simulink model "localizeUsingLidar"  (R2023b)
settings: Solver=VariableStepAuto  StartTime=0.0  StopTime=28.964  RelTol=1e-3
PreLoadFcn:
  | data = load('ReferencePathForward.mat');
  | 
  | refPosesX = data.ReferencePathForward.refPosesX;
  | refPosesY = data.ReferencePathForward.refPosesY;
  | refPosesT = data.ReferencePathForward.refPosesT;
  | 
  | load('parkingLotPCMapPoints.mat','ptCloudMapPoints');
model workspace (MAT data in the model file):
  ndtMap = pcmapndt
  ndtMap.any.SelectedSubmap = [-73.8227987289 40.1600699425 -29.3149013519 63.6737504005 0.110943684975 6.5344303928]
  ndtMap.any.XLimits = [-73.8227987289 40.1600699425]
  ndtMap.any.YLimits = [-29.3149013519 63.6737504005]
  ndtMap.any.ZLimits = [0.110943684975 6.5344303928]
  ndtMap.any.VoxelSize = 1
  ndtMap.any.VoxelMean = [-5.69730867658 -5.01883643014 -68.9383283343 -43.7471444266 11.2284455981 12.0427000258 13.2013916016 14.026733126 -69.7659169977 -45.9612937927 -43.6656163534 -18.7063802083 ... (31146 elements, 10382x3)]
  ndtMap.any.VoxelCovariance = [0.0677527841433 0.0204767959446 0.0010976444077 0.0204767959445 0.0285064886293 0.00050731343504 0.0010976444077 0.000507313435039 0.000784462408784 0.0377123915766 -0.00599493818508 0.000197123956374 ... (93438 elements, 3x3x10382)]
  ndtMap.any.VoxelInverseCovariance = [19.1019935486 -13.3999087348 -18.0623602948 -13.3999087348 44.8881032169 -10.2796550333 -18.0623602948 -10.2796550332 1306.67963741 55.6473126486 182.683156062 -17.3445014094 ... (93438 elements, 3x3x10382)]
  ndtMap.any.VoxelNumPoints = [7 7 7 7 7 9 20 14 11 10 6 12 ... (10382 elements, 10382x1)]
  ndtMap.any.Version = 1
undefined symbols (not defined in the file or in its folder): ptCloudMapPoints
libraries: sim3dautolib x36, sim3dphyssensorlib x1, sim3dlib x1
settings Model: Creator=The MathWorks, Inc.  LastModifiedBy=mahi1
settings SolverCC: AlgebraicLoopSolver=TrustRegion  MaxZcPerStep=1
settings DebuggingCC: UnconnectedInputMsg=warning  UnconnectedOutputMsg=warning  UnconnectedLineMsg=warning
settings ModelReferenceCC: EnableRefExpFcnMdlSchedulingChecks=on
settings RTWCC: DLArmComputeVersion=19.05

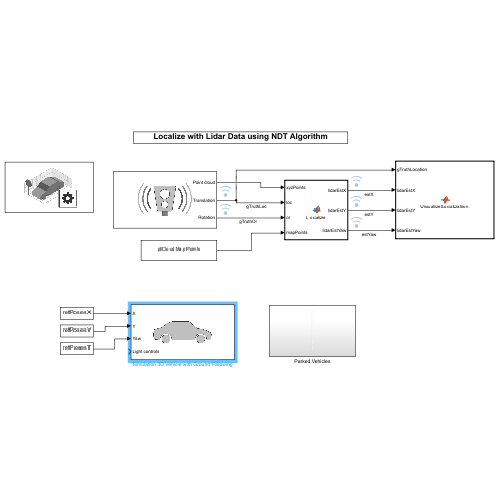
[thumbnail: Simulink's stored preview of the top-level diagram]
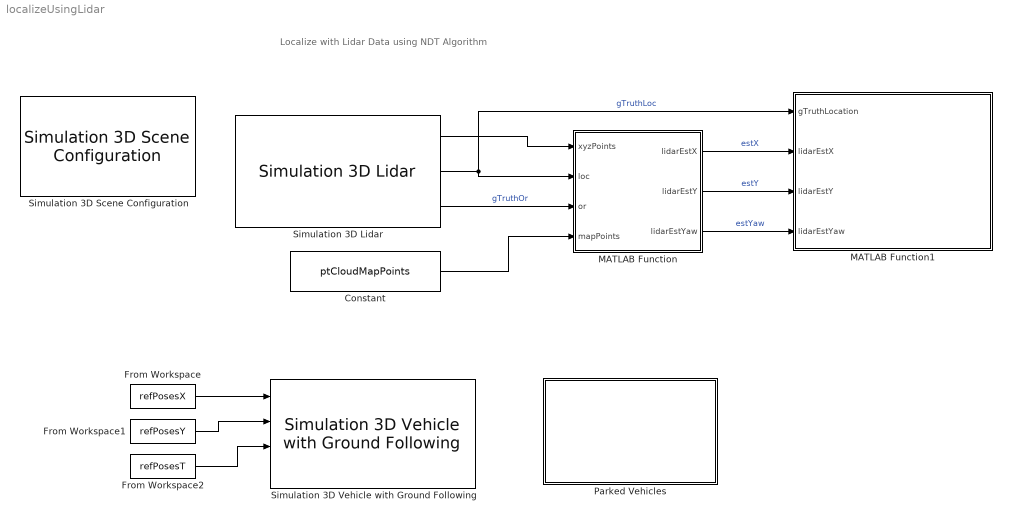
== system localizeUsingLidar ==
  note: Localize with Lidar Data using NDT Algorithm
  Constant : Constant  Value=ptCloudMapPoints
  From Workspace : FromWorkspace  VariableName=refPosesX  OutputAfterFinalValue=Holding final value
  From Workspace1 : FromWorkspace  VariableName=refPosesY  OutputAfterFinalValue=Holding final value
  From Workspace2 : FromWorkspace  VariableName=refPosesT  OutputAfterFinalValue=Holding final value
  MATLAB Function : MATLAB Function  TreatAsAtomicUnit=on
  MATLAB Function1 : MATLAB Function  StopFcn=|  TreatAsAtomicUnit=on
      | % Find figure by name
      | viewerFigure = findall(groot, 'type', 'figure', ...
      |     'name','Scene Map Display');
      | 
      | % Close figure
      | if ~isempty(viewerFigure)
      |     viewerFigure = viewerFigure(end);
      |     if isvalid(viewerFigure)
      |         close(viewerFigure);
      |     end
      | end
  Parked Vehicles : Subsystem
  Simulation 3D Lidar : sim3dphyssensorlib/Simulation 3D Lidar  Priority=1  sensorTag=Sim3dSensor1  sensorId=1  sensorName=Sim3dSensor1  vehTagList={'Scene Origin';'SimulinkVehicle1';'SimulinkVehicle10';'SimulinkVehicle11';'SimulinkVehicle12';'SimulinkVehicle13';'SimulinkVehicle14';'SimulinkVehicle15';'SimulinkVehicle16';'SimulinkVehicle17';'SimulinkVehicle18';'SimulinkVehicle19';'SimulinkVehicle2';'SimulinkVehicle20';'SimulinkVehicle21';'SimulinkVehicle22';'SimulinkVehicle23';'SimulinkVehicle24';'SimulinkVehicle25';'SimulinkVehicle26';'SimulinkVehicle27';'SimulinkVehicle28';'SimulinkVehicle29';'SimulinkVehicle3';'SimulinkVehicle30';'SimulinkVehicle31';'SimulinkVehicle32';'SimulinkVehicle33';'SimulinkVehicle34';'SimulinkVehicle35';'SimulinkVehicle36';'SimulinkVehicle4';'SimulinkVehicle5';'SimulinkVehicle6';'SimulinkVehicle7';'SimulinkVehicle8';'SimulinkVehicle9'}  vehTag=SimulinkVehicle1  mountLoc=Roof center  offsetFlag=off  tmountOffset=[0, 0, 0]  rmountOffset=[0, 0, 0]  DetectionRange=90  RangeResolution=0.002  VerticalFOV=40  VerticalResolution=1.25  HorizontalFOV=360  HorizontalResolution=0.332409972299169  DistanceOutportEnabled=off  ReflectivityOutportEnabled=off  SemanticOutportEnabled=off  TransformOutportEnabled=on  SampleTime=0.1  mountPoint=[-0.25 0 1.57000005245209]  mountOrientation=[0 0 0]  aMode=3  ID=1
      settings: LibrarySourceBlock=drivingsim3d/Simulation 3D Lidar
  Simulation 3D Scene Configuration : sim3dlib/Simulation 3D Scene Configuration  Priority=0  ProjectFormat=Default Scenes  SceneDesc=Large parking lot  ProjectName=D:\Matlab\toolbox\shared\sim3d_projects\automotive_project_windows\UE\WindowsNoEditor\VehicleSimulation.exe  ScenePath=/Game/Maps/HwStrght  EnableOpenDRIVE=off  vehTagList={'Scene Origin';'SimulinkVehicle1';'SimulinkVehicle10';'SimulinkVehicle11';'SimulinkVehicle12';'SimulinkVehicle13';'SimulinkVehicle14';'SimulinkVehicle15';'SimulinkVehicle16';'SimulinkVehicle17';'SimulinkVehicle18';'SimulinkVehicle19';'SimulinkVehicle2';'SimulinkVehicle20';'SimulinkVehicle21';'SimulinkVehicle22';'SimulinkVehicle23';'SimulinkVehicle24';'SimulinkVehicle25';'SimulinkVehicle26';'SimulinkVehicle27';'SimulinkVehicle28';'SimulinkVehicle29';'SimulinkVehicle3';'SimulinkVehicle30';'SimulinkVehicle31';'SimulinkVehicle32';'SimulinkVehicle33';'SimulinkVehicle34';'SimulinkVehicle35';'SimulinkVehicle36';'SimulinkVehicle4';'SimulinkVehicle5';'SimulinkVehicle6';'SimulinkVehicle7';'SimulinkVehicle8';'SimulinkVehicle9'}  vehTag=SimulinkVehicle1  FreeCameraInitialTranslation=[0, 0, 0]  FreeCameraDefaultInitialTranslation=[-6, 0, 2]  FreeCameraInitialRotation=[0, 0, 0]  FreeCameraDefaultInitialRotation=[0, -15, 0]  OpVisEn=off  Ts=0.02  EnableWindow=on  EnableRemoteAccess=off  EnableWeather=off  SunAltitude=40.0  SunAzimuth=90  clouds=10  wind=1  fog=0  rain=0  EnableGeospatial=off  OriginHeight=200  OriginLatitude=40.744652  OriginLongitude=-73.988864  MapStyle=Aerial  AdditionalAssetIDs=[]  UseAdvancedSunSky=off  SolarTime=11  TimeZone=-5  Day=21  Month=9  Year=2022  UseDaylightSavingTime=on  DSTStartDay=10  DSTStartMonth=3  DSTEndDay=3  DSTEndMonth=11  DSTSwitchHour=2  sensorTag=MainCamera2  sensorId=2  sensorName=MainCamera2  mountLoc=Origin  offsetFlag=off  tmountOffset=[0, 0, 0]  rmountOffset=[0, 0, 0]  HorizontalResolution=1280  VerticalResolution=720  HorizontalFOV=60  mountPoint=[0 0 0]  mountOrientation=[0 0 0]  aMode=3  ID=2  GeoTrigger=Inactive
      settings: LibrarySourceBlock=drivingsim3d/Simulation 3D Scene Configuration
  Simulation 3D Vehicle with Ground Following : sim3dautolib/Simulation 3D Vehicle with Ground Following  Priority=-1  PassVehMesh=Hatchback  MeshPath=/MathWorksSimulation/Vehicles/Muscle/Meshes/SK_MuscleCar.SK_MuscleCar  TrackWidth=1.9  WheelBase=3  WheelRadius=0.35  VehColor=Red  InitialPos=[refPosesX(1,2), refPosesY(1,2), 0]  InitialRot=[0, 0, refPosesT(1,2)]  ActorName=SimulinkVehicle1  SampleTime=-1  ActorType=SimulinkVehicle  ID=1  aMode=3  ActorTag=SimulinkVehicle1  CoordinateScheme=ISO  VehLightsControl=on  HeadlightColor=[ 1, 1, 1 ]  HighBeamIntensity=100000  LowBeamIntensity=60000  HighBeamConeAngle=70  LowBeamConeAngle=70  LeftHeadlightOrientation=[ 0, 0 ]  RightHeadlightOrientation=[ 0, 0 ]  BrakelightIntensity=5000  ReverselightIntensity=5000  SignallightIntensity=5000  SignallightPeriod=1  SignalPulseWidth=50  TransformOutportEnabled=off
      settings: LibrarySourceBlock=drivingsim3d/Simulation 3D Vehicle with Ground Following
  wires:
  From Workspace2/1 -> Simulation 3D Vehicle with Ground Following/3
  From Workspace/1 -> Simulation 3D Vehicle with Ground Following/1
  From Workspace1/1 -> Simulation 3D Vehicle with Ground Following/2
  Simulation 3D Lidar/1 -> MATLAB Function/1(xyzPoints)
  MATLAB Function/1(lidarEstX) -> MATLAB Function1/2(lidarEstX)  "estX"
  MATLAB Function/3(lidarEstYaw) -> MATLAB Function1/4(lidarEstYaw)  "estYaw"
  MATLAB Function/2(lidarEstY) -> MATLAB Function1/3(lidarEstY)  "estY"
  Simulation 3D Lidar/2 -> MATLAB Function1/1(gTruthLocation), MATLAB Function/2(loc)  "gTruthLoc"
  Simulation 3D Lidar/3 -> MATLAB Function/3(or)  "gTruthOr"
  Constant/1 -> MATLAB Function/4(mapPoints)

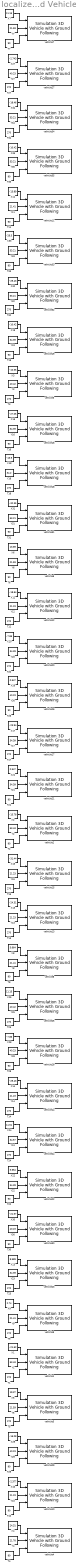
== system localizeUsingLidar/Parked Vehicles ==
  T{1,3,5,9,12..15,17..18,20,23..25,27,32,34} (17 alike) : Constant  Value=270
  T{2,4,6..8,10..11,16,19,21..22,26,28..31,33,35} (18 alike) : Constant  Value=90
  X1 : Constant  Value=-21.62
  X10 : Constant  Value=-2.377
  X11 : Constant  Value=-13.89
  X12 : Constant  Value=-18.64
  X13 : Constant  Value=-24.31
  X14 : Constant  Value=-29.43
  X15 : Constant  Value=-31.44
  X16 : Constant  Value=-27.05
  X17 : Constant  Value=-23.94
  X18 : Constant  Value=-15.9
  X19 : Constant  Value=-10.42
  X2 : Constant  Value=-15.78
  X20 : Constant  Value=-7.86
  X21 : Constant  Value=0.547
  X22 : Constant  Value=5.664
  X23 : Constant  Value=8.589
  X24 : Constant  Value=11.51
  X25 : Constant  Value=11.15
  X26 : Constant  Value=0.547
  X27 : Constant  Value=-2.743
  X28 : Constant  Value=-7.86
  X29 : Constant  Value=-16.08
  X3 : Constant  Value=-10.55
  X30 : Constant  Value=-21.57
  X31 : Constant  Value=-32.35
  X32 : Constant  Value=-29.43
  X33 : Constant  Value=-26.5
  X34 : Constant  Value=-18.46
  X35 : Constant  Value=-10.42
  X4 : Constant  Value=24.31
  X5 : Constant  Value=19.37
  X6 : Constant  Value=13.89
  X7 : Constant  Value=11.15
  X8 : Constant  Value=5.664
  X9 : Constant  Value=2.74
  Y1 : Constant  Value=53.43
  Y{10,12..15} (5 alike) : Constant  Value=21.23
  Y11 : Constant  Value=21.41
  Y{16..17,19..23} (7 alike) : Constant  Value=34.39
  Y18 : Constant  Value=34.2
  Y2 : Constant  Value=53.43
  Y24 : Constant  Value=34.57
  Y25 : Constant  Value=40.42
  Y{26..30} (5 alike) : Constant  Value=40.23
  Y3 : Constant  Value=40.42
  Y{31..35} (5 alike) : Constant  Value=53.21
  Y4 : Constant  Value=21.78
  Y5 : Constant  Value=21.59
  Y6 : Constant  Value=21.59
  Y7 : Constant  Value=21.59
  Y8 : Constant  Value=21.41
  Y9 : Constant  Value=21.41
  vehicle1 : sim3dautolib/Simulation 3D Vehicle with Ground Following  Priority=-1  PassVehMesh=Small pickup truck  MeshPath=/MathWorksSimulation/Vehicles/Muscle/Meshes/SK_MuscleCar.SK_MuscleCar  TrackWidth=1.9  WheelBase=3  WheelRadius=0.35  VehColor=Silver  InitialPos=[-21.62 53.43 0]  InitialRot=[0 0 270]  ActorName=SimulinkVehicle2  SampleTime=-1  ActorType=SimulinkVehicle  ID=2  aMode=3  ActorTag=SimulinkVehicle2  CoordinateScheme=ISO  VehLightsControl=off  HeadlightColor=[ 1, 1, 1 ]  HighBeamIntensity=100000  LowBeamIntensity=60000  HighBeamConeAngle=70  LowBeamConeAngle=70  LeftHeadlightOrientation=[ 0, 0 ]  RightHeadlightOrientation=[ 0, 0 ]  BrakelightIntensity=500  ReverselightIntensity=500  SignallightIntensity=500  SignallightPeriod=1  SignalPulseWidth=50  TransformOutportEnabled=off
      settings: LibrarySourceBlock=drivingsim3d/Simulation 3D Vehicle with Ground Following
  vehicle10 : sim3dautolib/Simulation 3D Vehicle with Ground Following  Priority=-1  PassVehMesh=Small pickup truck  MeshPath=/MathWorksSimulation/Vehicles/Muscle/Meshes/SK_MuscleCar.SK_MuscleCar  TrackWidth=1.9  WheelBase=3  WheelRadius=0.35  VehColor=Orange  InitialPos=[-2.377 21.23 0]  InitialRot=[0 0 90]  ActorName=SimulinkVehicle11  SampleTime=-1  ActorType=SimulinkVehicle  ID=11  aMode=3  ActorTag=SimulinkVehicle11  CoordinateScheme=ISO  VehLightsControl=off  HeadlightColor=[ 1, 1, 1 ]  HighBeamIntensity=100000  LowBeamIntensity=60000  HighBeamConeAngle=70  LowBeamConeAngle=70  LeftHeadlightOrientation=[ 0, 0 ]  RightHeadlightOrientation=[ 0, 0 ]  BrakelightIntensity=500  ReverselightIntensity=500  SignallightIntensity=500  SignallightPeriod=1  SignalPulseWidth=50  TransformOutportEnabled=off
      settings: LibrarySourceBlock=drivingsim3d/Simulation 3D Vehicle with Ground Following
  vehicle11 : sim3dautolib/Simulation 3D Vehicle with Ground Following  Priority=-1  PassVehMesh=Hatchback  MeshPath=/MathWorksSimulation/Vehicles/Muscle/Meshes/SK_MuscleCar.SK_MuscleCar  TrackWidth=1.9  WheelBase=3  WheelRadius=0.35  VehColor=Green  InitialPos=[-13.89 21.41 0]  InitialRot=[0 0 90]  ActorName=SimulinkVehicle12  SampleTime=-1  ActorType=SimulinkVehicle  ID=12  aMode=3  ActorTag=SimulinkVehicle12  CoordinateScheme=ISO  VehLightsControl=off  HeadlightColor=[ 1, 1, 1 ]  HighBeamIntensity=100000  LowBeamIntensity=60000  HighBeamConeAngle=70  LowBeamConeAngle=70  LeftHeadlightOrientation=[ 0, 0 ]  RightHeadlightOrientation=[ 0, 0 ]  BrakelightIntensity=500  ReverselightIntensity=500  SignallightIntensity=500  SignallightPeriod=1  SignalPulseWidth=50  TransformOutportEnabled=off
      settings: LibrarySourceBlock=drivingsim3d/Simulation 3D Vehicle with Ground Following
  vehicle12 : sim3dautolib/Simulation 3D Vehicle with Ground Following  Priority=-1  PassVehMesh=Small pickup truck  MeshPath=/MathWorksSimulation/Vehicles/Muscle/Meshes/SK_MuscleCar.SK_MuscleCar  TrackWidth=1.9  WheelBase=3  WheelRadius=0.35  VehColor=Green  InitialPos=[-18.64 21.23 0]  InitialRot=[0 0 270]  ActorName=SimulinkVehicle13  SampleTime=-1  ActorType=SimulinkVehicle  ID=13  aMode=3  ActorTag=SimulinkVehicle13  CoordinateScheme=ISO  VehLightsControl=off  HeadlightColor=[ 1, 1, 1 ]  HighBeamIntensity=100000  LowBeamIntensity=60000  HighBeamConeAngle=70  LowBeamConeAngle=70  LeftHeadlightOrientation=[ 0, 0 ]  RightHeadlightOrientation=[ 0, 0 ]  BrakelightIntensity=500  ReverselightIntensity=500  SignallightIntensity=500  SignallightPeriod=1  SignalPulseWidth=50  TransformOutportEnabled=off
      settings: LibrarySourceBlock=drivingsim3d/Simulation 3D Vehicle with Ground Following
  vehicle13 : sim3dautolib/Simulation 3D Vehicle with Ground Following  Priority=-1  PassVehMesh=Small pickup truck  MeshPath=/MathWorksSimulation/Vehicles/Muscle/Meshes/SK_MuscleCar.SK_MuscleCar  TrackWidth=1.9  WheelBase=3  WheelRadius=0.35  VehColor=Black  InitialPos=[-24.31 21.23 0]  InitialRot=[0 0 270]  ActorName=SimulinkVehicle14  SampleTime=-1  ActorType=SimulinkVehicle  ID=14  aMode=3  ActorTag=SimulinkVehicle14  CoordinateScheme=ISO  VehLightsControl=off  HeadlightColor=[ 1, 1, 1 ]  HighBeamIntensity=100000  LowBeamIntensity=60000  HighBeamConeAngle=70  LowBeamConeAngle=70  LeftHeadlightOrientation=[ 0, 0 ]  RightHeadlightOrientation=[ 0, 0 ]  BrakelightIntensity=500  ReverselightIntensity=500  SignallightIntensity=500  SignallightPeriod=1  SignalPulseWidth=50  TransformOutportEnabled=off
      settings: LibrarySourceBlock=drivingsim3d/Simulation 3D Vehicle with Ground Following
  vehicle14 : sim3dautolib/Simulation 3D Vehicle with Ground Following  Priority=-1  PassVehMesh=Sport utility vehicle  MeshPath=/MathWorksSimulation/Vehicles/Muscle/Meshes/SK_MuscleCar.SK_MuscleCar  TrackWidth=1.9  WheelBase=3  WheelRadius=0.35  VehColor=Black  InitialPos=[-29.43 21.23 0]  InitialRot=[0 0 270]  ActorName=SimulinkVehicle15  SampleTime=-1  ActorType=SimulinkVehicle  ID=15  aMode=3  ActorTag=SimulinkVehicle15  CoordinateScheme=ISO  VehLightsControl=off  HeadlightColor=[ 1, 1, 1 ]  HighBeamIntensity=100000  LowBeamIntensity=60000  HighBeamConeAngle=70  LowBeamConeAngle=70  LeftHeadlightOrientation=[ 0, 0 ]  RightHeadlightOrientation=[ 0, 0 ]  BrakelightIntensity=500  ReverselightIntensity=500  SignallightIntensity=500  SignallightPeriod=1  SignalPulseWidth=50  TransformOutportEnabled=off
      settings: LibrarySourceBlock=drivingsim3d/Simulation 3D Vehicle with Ground Following
  vehicle15 : sim3dautolib/Simulation 3D Vehicle with Ground Following  Priority=-1  PassVehMesh=Small pickup truck  MeshPath=/MathWorksSimulation/Vehicles/Muscle/Meshes/SK_MuscleCar.SK_MuscleCar  TrackWidth=1.9  WheelBase=3  WheelRadius=0.35  VehColor=Silver  InitialPos=[-31.44 21.23 0]  InitialRot=[0 0 270]  ActorName=SimulinkVehicle16  SampleTime=-1  ActorType=SimulinkVehicle  ID=16  aMode=3  ActorTag=SimulinkVehicle16  CoordinateScheme=ISO  VehLightsControl=off  HeadlightColor=[ 1, 1, 1 ]  HighBeamIntensity=100000  LowBeamIntensity=60000  HighBeamConeAngle=70  LowBeamConeAngle=70  LeftHeadlightOrientation=[ 0, 0 ]  RightHeadlightOrientation=[ 0, 0 ]  BrakelightIntensity=500  ReverselightIntensity=500  SignallightIntensity=500  SignallightPeriod=1  SignalPulseWidth=50  TransformOutportEnabled=off
      settings: LibrarySourceBlock=drivingsim3d/Simulation 3D Vehicle with Ground Following
  vehicle16 : sim3dautolib/Simulation 3D Vehicle with Ground Following  Priority=-1  PassVehMesh=Hatchback  MeshPath=/MathWorksSimulation/Vehicles/Muscle/Meshes/SK_MuscleCar.SK_MuscleCar  TrackWidth=1.9  WheelBase=3  WheelRadius=0.35  VehColor=Yellow  InitialPos=[-27.05 34.39 0]  InitialRot=[0 0 90]  ActorName=SimulinkVehicle17  SampleTime=-1  ActorType=SimulinkVehicle  ID=17  aMode=3  ActorTag=SimulinkVehicle17  CoordinateScheme=ISO  VehLightsControl=off  HeadlightColor=[ 1, 1, 1 ]  HighBeamIntensity=100000  LowBeamIntensity=60000  HighBeamConeAngle=70  LowBeamConeAngle=70  LeftHeadlightOrientation=[ 0, 0 ]  RightHeadlightOrientation=[ 0, 0 ]  BrakelightIntensity=500  ReverselightIntensity=500  SignallightIntensity=500  SignallightPeriod=1  SignalPulseWidth=50  TransformOutportEnabled=off
      settings: LibrarySourceBlock=drivingsim3d/Simulation 3D Vehicle with Ground Following
  vehicle17 : sim3dautolib/Simulation 3D Vehicle with Ground Following  Priority=-1  PassVehMesh=Sport utility vehicle  MeshPath=/MathWorksSimulation/Vehicles/Muscle/Meshes/SK_MuscleCar.SK_MuscleCar  TrackWidth=1.9  WheelBase=3  WheelRadius=0.35  VehColor=Black  InitialPos=[-23.94 34.39 0]  InitialRot=[0 0 270]  ActorName=SimulinkVehicle18  SampleTime=-1  ActorType=SimulinkVehicle  ID=18  aMode=3  ActorTag=SimulinkVehicle18  CoordinateScheme=ISO  VehLightsControl=off  HeadlightColor=[ 1, 1, 1 ]  HighBeamIntensity=100000  LowBeamIntensity=60000  HighBeamConeAngle=70  LowBeamConeAngle=70  LeftHeadlightOrientation=[ 0, 0 ]  RightHeadlightOrientation=[ 0, 0 ]  BrakelightIntensity=500  ReverselightIntensity=500  SignallightIntensity=500  SignallightPeriod=1  SignalPulseWidth=50  TransformOutportEnabled=off
      settings: LibrarySourceBlock=drivingsim3d/Simulation 3D Vehicle with Ground Following
  vehicle18 : sim3dautolib/Simulation 3D Vehicle with Ground Following  Priority=-1  PassVehMesh=Small pickup truck  MeshPath=/MathWorksSimulation/Vehicles/Muscle/Meshes/SK_MuscleCar.SK_MuscleCar  TrackWidth=1.9  WheelBase=3  WheelRadius=0.35  VehColor=Black  InitialPos=[-15.9 34.2 0]  InitialRot=[0 0 270]  ActorName=SimulinkVehicle19  SampleTime=-1  ActorType=SimulinkVehicle  ID=19  aMode=3  ActorTag=SimulinkVehicle19  CoordinateScheme=ISO  VehLightsControl=off  HeadlightColor=[ 1, 1, 1 ]  HighBeamIntensity=100000  LowBeamIntensity=60000  HighBeamConeAngle=70  LowBeamConeAngle=70  LeftHeadlightOrientation=[ 0, 0 ]  RightHeadlightOrientation=[ 0, 0 ]  BrakelightIntensity=500  ReverselightIntensity=500  SignallightIntensity=500  SignallightPeriod=1  SignalPulseWidth=50  TransformOutportEnabled=off
      settings: LibrarySourceBlock=drivingsim3d/Simulation 3D Vehicle with Ground Following
  vehicle19 : sim3dautolib/Simulation 3D Vehicle with Ground Following  Priority=-1  PassVehMesh=Sedan  MeshPath=/MathWorksSimulation/Vehicles/Muscle/Meshes/SK_MuscleCar.SK_MuscleCar  TrackWidth=1.9  WheelBase=3  WheelRadius=0.35  VehColor=Orange  InitialPos=[-10.42 34.39 0]  InitialRot=[0 0 90]  ActorName=SimulinkVehicle20  SampleTime=-1  ActorType=SimulinkVehicle  ID=20  aMode=3  ActorTag=SimulinkVehicle20  CoordinateScheme=ISO  VehLightsControl=off  HeadlightColor=[ 1, 1, 1 ]  HighBeamIntensity=100000  LowBeamIntensity=60000  HighBeamConeAngle=70  LowBeamConeAngle=70  LeftHeadlightOrientation=[ 0, 0 ]  RightHeadlightOrientation=[ 0, 0 ]  BrakelightIntensity=500  ReverselightIntensity=500  SignallightIntensity=500  SignallightPeriod=1  SignalPulseWidth=50  TransformOutportEnabled=off
      settings: LibrarySourceBlock=drivingsim3d/Simulation 3D Vehicle with Ground Following
  vehicle2 : sim3dautolib/Simulation 3D Vehicle with Ground Following  Priority=-1  PassVehMesh=Small pickup truck  MeshPath=/MathWorksSimulation/Vehicles/Muscle/Meshes/SK_MuscleCar.SK_MuscleCar  TrackWidth=1.9  WheelBase=3  WheelRadius=0.35  VehColor=Black  InitialPos=[-15.78 53.43 0]  InitialRot=[0 0 90]  ActorName=SimulinkVehicle3  SampleTime=-1  ActorType=SimulinkVehicle  ID=3  aMode=3  ActorTag=SimulinkVehicle3  CoordinateScheme=ISO  VehLightsControl=off  HeadlightColor=[ 1, 1, 1 ]  HighBeamIntensity=100000  LowBeamIntensity=60000  HighBeamConeAngle=70  LowBeamConeAngle=70  LeftHeadlightOrientation=[ 0, 0 ]  RightHeadlightOrientation=[ 0, 0 ]  BrakelightIntensity=500  ReverselightIntensity=500  SignallightIntensity=500  SignallightPeriod=1  SignalPulseWidth=50  TransformOutportEnabled=off
      settings: LibrarySourceBlock=drivingsim3d/Simulation 3D Vehicle with Ground Following
  vehicle20 : sim3dautolib/Simulation 3D Vehicle with Ground Following  Priority=-1  PassVehMesh=Small pickup truck  MeshPath=/MathWorksSimulation/Vehicles/Muscle/Meshes/SK_MuscleCar.SK_MuscleCar  TrackWidth=1.9  WheelBase=3  WheelRadius=0.35  VehColor=Red  InitialPos=[-7.86 34.39 0]  InitialRot=[0 0 270]  ActorName=SimulinkVehicle21  SampleTime=-1  ActorType=SimulinkVehicle  ID=21  aMode=3  ActorTag=SimulinkVehicle21  CoordinateScheme=ISO  VehLightsControl=off  HeadlightColor=[ 1, 1, 1 ]  HighBeamIntensity=100000  LowBeamIntensity=60000  HighBeamConeAngle=70  LowBeamConeAngle=70  LeftHeadlightOrientation=[ 0, 0 ]  RightHeadlightOrientation=[ 0, 0 ]  BrakelightIntensity=500  ReverselightIntensity=500  SignallightIntensity=500  SignallightPeriod=1  SignalPulseWidth=50  TransformOutportEnabled=off
      settings: LibrarySourceBlock=drivingsim3d/Simulation 3D Vehicle with Ground Following
  vehicle21 : sim3dautolib/Simulation 3D Vehicle with Ground Following  Priority=-1  PassVehMesh=Sedan  MeshPath=/MathWorksSimulation/Vehicles/Muscle/Meshes/SK_MuscleCar.SK_MuscleCar  TrackWidth=1.9  WheelBase=3  WheelRadius=0.35  VehColor=Green  InitialPos=[0.547 34.39 0]  InitialRot=[0 0 90]  ActorName=SimulinkVehicle22  SampleTime=-1  ActorType=SimulinkVehicle  ID=22  aMode=3  ActorTag=SimulinkVehicle22  CoordinateScheme=ISO  VehLightsControl=off  HeadlightColor=[ 1, 1, 1 ]  HighBeamIntensity=100000  LowBeamIntensity=60000  HighBeamConeAngle=70  LowBeamConeAngle=70  LeftHeadlightOrientation=[ 0, 0 ]  RightHeadlightOrientation=[ 0, 0 ]  BrakelightIntensity=500  ReverselightIntensity=500  SignallightIntensity=500  SignallightPeriod=1  SignalPulseWidth=50  TransformOutportEnabled=off
      settings: LibrarySourceBlock=drivingsim3d/Simulation 3D Vehicle with Ground Following
  vehicle22 : sim3dautolib/Simulation 3D Vehicle with Ground Following  Priority=-1  PassVehMesh=Hatchback  MeshPath=/MathWorksSimulation/Vehicles/Muscle/Meshes/SK_MuscleCar.SK_MuscleCar  TrackWidth=1.9  WheelBase=3  WheelRadius=0.35  VehColor=White  InitialPos=[5.664 34.39 0]  InitialRot=[0 0 90]  ActorName=SimulinkVehicle23  SampleTime=-1  ActorType=SimulinkVehicle  ID=23  aMode=3  ActorTag=SimulinkVehicle23  CoordinateScheme=ISO  VehLightsControl=off  HeadlightColor=[ 1, 1, 1 ]  HighBeamIntensity=100000  LowBeamIntensity=60000  HighBeamConeAngle=70  LowBeamConeAngle=70  LeftHeadlightOrientation=[ 0, 0 ]  RightHeadlightOrientation=[ 0, 0 ]  BrakelightIntensity=500  ReverselightIntensity=500  SignallightIntensity=500  SignallightPeriod=1  SignalPulseWidth=50  TransformOutportEnabled=off
      settings: LibrarySourceBlock=drivingsim3d/Simulation 3D Vehicle with Ground Following
  vehicle23 : sim3dautolib/Simulation 3D Vehicle with Ground Following  Priority=-1  PassVehMesh=Small pickup truck  MeshPath=/MathWorksSimulation/Vehicles/Muscle/Meshes/SK_MuscleCar.SK_MuscleCar  TrackWidth=1.9  WheelBase=3  WheelRadius=0.35  VehColor=Yellow  InitialPos=[8.589 34.39 0]  InitialRot=[0 0 270]  ActorName=SimulinkVehicle24  SampleTime=-1  ActorType=SimulinkVehicle  ID=24  aMode=3  ActorTag=SimulinkVehicle24  CoordinateScheme=ISO  VehLightsControl=off  HeadlightColor=[ 1, 1, 1 ]  HighBeamIntensity=100000  LowBeamIntensity=60000  HighBeamConeAngle=70  LowBeamConeAngle=70  LeftHeadlightOrientation=[ 0, 0 ]  RightHeadlightOrientation=[ 0, 0 ]  BrakelightIntensity=500  ReverselightIntensity=500  SignallightIntensity=500  SignallightPeriod=1  SignalPulseWidth=50  TransformOutportEnabled=off
      settings: LibrarySourceBlock=drivingsim3d/Simulation 3D Vehicle with Ground Following
  vehicle24 : sim3dautolib/Simulation 3D Vehicle with Ground Following  Priority=-1  PassVehMesh=Small pickup truck  MeshPath=/MathWorksSimulation/Vehicles/Muscle/Meshes/SK_MuscleCar.SK_MuscleCar  TrackWidth=1.9  WheelBase=3  WheelRadius=0.35  VehColor=Blue  InitialPos=[11.51 34.57 0]  InitialRot=[0 0 270]  ActorName=SimulinkVehicle25  SampleTime=-1  ActorType=SimulinkVehicle  ID=25  aMode=3  ActorTag=SimulinkVehicle25  CoordinateScheme=ISO  VehLightsControl=off  HeadlightColor=[ 1, 1, 1 ]  HighBeamIntensity=100000  LowBeamIntensity=60000  HighBeamConeAngle=70  LowBeamConeAngle=70  LeftHeadlightOrientation=[ 0, 0 ]  RightHeadlightOrientation=[ 0, 0 ]  BrakelightIntensity=500  ReverselightIntensity=500  SignallightIntensity=500  SignallightPeriod=1  SignalPulseWidth=50  TransformOutportEnabled=off
      settings: LibrarySourceBlock=drivingsim3d/Simulation 3D Vehicle with Ground Following
  vehicle25 : sim3dautolib/Simulation 3D Vehicle with Ground Following  Priority=-1  PassVehMesh=Sedan  MeshPath=/MathWorksSimulation/Vehicles/Muscle/Meshes/SK_MuscleCar.SK_MuscleCar  TrackWidth=1.9  WheelBase=3  WheelRadius=0.35  VehColor=Orange  InitialPos=[11.15 40.42 0]  InitialRot=[0 0 270]  ActorName=SimulinkVehicle26  SampleTime=-1  ActorType=SimulinkVehicle  ID=26  aMode=3  ActorTag=SimulinkVehicle26  CoordinateScheme=ISO  VehLightsControl=off  HeadlightColor=[ 1, 1, 1 ]  HighBeamIntensity=100000  LowBeamIntensity=60000  HighBeamConeAngle=70  LowBeamConeAngle=70  LeftHeadlightOrientation=[ 0, 0 ]  RightHeadlightOrientation=[ 0, 0 ]  BrakelightIntensity=500  ReverselightIntensity=500  SignallightIntensity=500  SignallightPeriod=1  SignalPulseWidth=50  TransformOutportEnabled=off
      settings: LibrarySourceBlock=drivingsim3d/Simulation 3D Vehicle with Ground Following
  vehicle26 : sim3dautolib/Simulation 3D Vehicle with Ground Following  Priority=-1  PassVehMesh=Sedan  MeshPath=/MathWorksSimulation/Vehicles/Muscle/Meshes/SK_MuscleCar.SK_MuscleCar  TrackWidth=1.9  WheelBase=3  WheelRadius=0.35  VehColor=Silver  InitialPos=[0.547 40.23 0]  InitialRot=[0 0 90]  ActorName=SimulinkVehicle27  SampleTime=-1  ActorType=SimulinkVehicle  ID=27  aMode=3  ActorTag=SimulinkVehicle27  CoordinateScheme=ISO  VehLightsControl=off  HeadlightColor=[ 1, 1, 1 ]  HighBeamIntensity=100000  LowBeamIntensity=60000  HighBeamConeAngle=70  LowBeamConeAngle=70  LeftHeadlightOrientation=[ 0, 0 ]  RightHeadlightOrientation=[ 0, 0 ]  BrakelightIntensity=500  ReverselightIntensity=500  SignallightIntensity=500  SignallightPeriod=1  SignalPulseWidth=50  TransformOutportEnabled=off
      settings: LibrarySourceBlock=drivingsim3d/Simulation 3D Vehicle with Ground Following
  vehicle27 : sim3dautolib/Simulation 3D Vehicle with Ground Following  Priority=-1  PassVehMesh=Sedan  MeshPath=/MathWorksSimulation/Vehicles/Muscle/Meshes/SK_MuscleCar.SK_MuscleCar  TrackWidth=1.9  WheelBase=3  WheelRadius=0.35  VehColor=Yellow  InitialPos=[-2.743 40.23 0]  InitialRot=[0 0 270]  ActorName=SimulinkVehicle28  SampleTime=-1  ActorType=SimulinkVehicle  ID=28  aMode=3  ActorTag=SimulinkVehicle28  CoordinateScheme=ISO  VehLightsControl=off  HeadlightColor=[ 1, 1, 1 ]  HighBeamIntensity=100000  LowBeamIntensity=60000  HighBeamConeAngle=70  LowBeamConeAngle=70  LeftHeadlightOrientation=[ 0, 0 ]  RightHeadlightOrientation=[ 0, 0 ]  BrakelightIntensity=500  ReverselightIntensity=500  SignallightIntensity=500  SignallightPeriod=1  SignalPulseWidth=50  TransformOutportEnabled=off
      settings: LibrarySourceBlock=drivingsim3d/Simulation 3D Vehicle with Ground Following
  vehicle28 : sim3dautolib/Simulation 3D Vehicle with Ground Following  Priority=-1  PassVehMesh=Muscle car  MeshPath=/MathWorksSimulation/Vehicles/Muscle/Meshes/SK_MuscleCar.SK_MuscleCar  TrackWidth=1.9  WheelBase=3  WheelRadius=0.35  VehColor=Blue  InitialPos=[-7.86 40.23 0]  InitialRot=[0 0 90]  ActorName=SimulinkVehicle29  SampleTime=-1  ActorType=SimulinkVehicle  ID=29  aMode=3  ActorTag=SimulinkVehicle29  CoordinateScheme=ISO  VehLightsControl=off  HeadlightColor=[ 1, 1, 1 ]  HighBeamIntensity=100000  LowBeamIntensity=60000  HighBeamConeAngle=70  LowBeamConeAngle=70  LeftHeadlightOrientation=[ 0, 0 ]  RightHeadlightOrientation=[ 0, 0 ]  BrakelightIntensity=500  ReverselightIntensity=500  SignallightIntensity=500  SignallightPeriod=1  SignalPulseWidth=50  TransformOutportEnabled=off
      settings: LibrarySourceBlock=drivingsim3d/Simulation 3D Vehicle with Ground Following
  vehicle29 : sim3dautolib/Simulation 3D Vehicle with Ground Following  Priority=-1  PassVehMesh=Sedan  MeshPath=/MathWorksSimulation/Vehicles/Muscle/Meshes/SK_MuscleCar.SK_MuscleCar  TrackWidth=1.9  WheelBase=3  WheelRadius=0.35  VehColor=Black  InitialPos=[-16.08 40.23 0]  InitialRot=[0 0 90]  ActorName=SimulinkVehicle30  SampleTime=-1  ActorType=SimulinkVehicle  ID=30  aMode=3  ActorTag=SimulinkVehicle30  CoordinateScheme=ISO  VehLightsControl=off  HeadlightColor=[ 1, 1, 1 ]  HighBeamIntensity=100000  LowBeamIntensity=60000  HighBeamConeAngle=70  LowBeamConeAngle=70  LeftHeadlightOrientation=[ 0, 0 ]  RightHeadlightOrientation=[ 0, 0 ]  BrakelightIntensity=500  ReverselightIntensity=500  SignallightIntensity=500  SignallightPeriod=1  SignalPulseWidth=50  TransformOutportEnabled=off
      settings: LibrarySourceBlock=drivingsim3d/Simulation 3D Vehicle with Ground Following
  vehicle3 : sim3dautolib/Simulation 3D Vehicle with Ground Following  Priority=-1  PassVehMesh=Hatchback  MeshPath=/MathWorksSimulation/Vehicles/Muscle/Meshes/SK_MuscleCar.SK_MuscleCar  TrackWidth=1.9  WheelBase=3  WheelRadius=0.35  VehColor=Yellow  InitialPos=[-10.55 40.42 0]  InitialRot=[0 0 270]  ActorName=SimulinkVehicle4  SampleTime=-1  ActorType=SimulinkVehicle  ID=4  aMode=3  ActorTag=SimulinkVehicle4  CoordinateScheme=ISO  VehLightsControl=off  HeadlightColor=[ 1, 1, 1 ]  HighBeamIntensity=100000  LowBeamIntensity=60000  HighBeamConeAngle=70  LowBeamConeAngle=70  LeftHeadlightOrientation=[ 0, 0 ]  RightHeadlightOrientation=[ 0, 0 ]  BrakelightIntensity=500  ReverselightIntensity=500  SignallightIntensity=500  SignallightPeriod=1  SignalPulseWidth=50  TransformOutportEnabled=off
      settings: LibrarySourceBlock=drivingsim3d/Simulation 3D Vehicle with Ground Following
  vehicle30 : sim3dautolib/Simulation 3D Vehicle with Ground Following  Priority=-1  PassVehMesh=Hatchback  MeshPath=/MathWorksSimulation/Vehicles/Muscle/Meshes/SK_MuscleCar.SK_MuscleCar  TrackWidth=1.9  WheelBase=3  WheelRadius=0.35  VehColor=White  InitialPos=[-21.57 40.23 0]  InitialRot=[0 0 90]  ActorName=SimulinkVehicle31  SampleTime=-1  ActorType=SimulinkVehicle  ID=31  aMode=3  ActorTag=SimulinkVehicle31  CoordinateScheme=ISO  VehLightsControl=off  HeadlightColor=[ 1, 1, 1 ]  HighBeamIntensity=100000  LowBeamIntensity=60000  HighBeamConeAngle=70  LowBeamConeAngle=70  LeftHeadlightOrientation=[ 0, 0 ]  RightHeadlightOrientation=[ 0, 0 ]  BrakelightIntensity=500  ReverselightIntensity=500  SignallightIntensity=500  SignallightPeriod=1  SignalPulseWidth=50  TransformOutportEnabled=off
      settings: LibrarySourceBlock=drivingsim3d/Simulation 3D Vehicle with Ground Following
  vehicle31 : sim3dautolib/Simulation 3D Vehicle with Ground Following  Priority=-1  PassVehMesh=Sedan  MeshPath=/MathWorksSimulation/Vehicles/Muscle/Meshes/SK_MuscleCar.SK_MuscleCar  TrackWidth=1.9  WheelBase=3  WheelRadius=0.35  VehColor=White  InitialPos=[-32.35 53.21 0]  InitialRot=[0 0 90]  ActorName=SimulinkVehicle32  SampleTime=-1  ActorType=SimulinkVehicle  ID=32  aMode=3  ActorTag=SimulinkVehicle32  CoordinateScheme=ISO  VehLightsControl=off  HeadlightColor=[ 1, 1, 1 ]  HighBeamIntensity=100000  LowBeamIntensity=60000  HighBeamConeAngle=70  LowBeamConeAngle=70  LeftHeadlightOrientation=[ 0, 0 ]  RightHeadlightOrientation=[ 0, 0 ]  BrakelightIntensity=500  ReverselightIntensity=500  SignallightIntensity=500  SignallightPeriod=1  SignalPulseWidth=50  TransformOutportEnabled=off
      settings: LibrarySourceBlock=drivingsim3d/Simulation 3D Vehicle with Ground Following
  vehicle32 : sim3dautolib/Simulation 3D Vehicle with Ground Following  Priority=-1  PassVehMesh=Hatchback  MeshPath=/MathWorksSimulation/Vehicles/Muscle/Meshes/SK_MuscleCar.SK_MuscleCar  TrackWidth=1.9  WheelBase=3  WheelRadius=0.35  VehColor=Blue  InitialPos=[-29.43 53.21 0]  InitialRot=[0 0 270]  ActorName=SimulinkVehicle33  SampleTime=-1  ActorType=SimulinkVehicle  ID=33  aMode=3  ActorTag=SimulinkVehicle33  CoordinateScheme=ISO  VehLightsControl=off  HeadlightColor=[ 1, 1, 1 ]  HighBeamIntensity=100000  LowBeamIntensity=60000  HighBeamConeAngle=70  LowBeamConeAngle=70  LeftHeadlightOrientation=[ 0, 0 ]  RightHeadlightOrientation=[ 0, 0 ]  BrakelightIntensity=500  ReverselightIntensity=500  SignallightIntensity=500  SignallightPeriod=1  SignalPulseWidth=50  TransformOutportEnabled=off
      settings: LibrarySourceBlock=drivingsim3d/Simulation 3D Vehicle with Ground Following
  vehicle33 : sim3dautolib/Simulation 3D Vehicle with Ground Following  Priority=-1  PassVehMesh=Muscle car  MeshPath=/MathWorksSimulation/Vehicles/Muscle/Meshes/SK_MuscleCar.SK_MuscleCar  TrackWidth=1.9  WheelBase=3  WheelRadius=0.35  VehColor=Orange  InitialPos=[-26.5 53.21 0]  InitialRot=[0 0 90]  ActorName=SimulinkVehicle34  SampleTime=-1  ActorType=SimulinkVehicle  ID=34  aMode=3  ActorTag=SimulinkVehicle34  CoordinateScheme=ISO  VehLightsControl=off  HeadlightColor=[ 1, 1, 1 ]  HighBeamIntensity=100000  LowBeamIntensity=60000  HighBeamConeAngle=70  LowBeamConeAngle=70  LeftHeadlightOrientation=[ 0, 0 ]  RightHeadlightOrientation=[ 0, 0 ]  BrakelightIntensity=500  ReverselightIntensity=500  SignallightIntensity=500  SignallightPeriod=1  SignalPulseWidth=50  TransformOutportEnabled=off
      settings: LibrarySourceBlock=drivingsim3d/Simulation 3D Vehicle with Ground Following
  vehicle34 : sim3dautolib/Simulation 3D Vehicle with Ground Following  Priority=-1  PassVehMesh=Hatchback  MeshPath=/MathWorksSimulation/Vehicles/Muscle/Meshes/SK_MuscleCar.SK_MuscleCar  TrackWidth=1.9  WheelBase=3  WheelRadius=0.35  VehColor=Orange  InitialPos=[-18.46 53.21 0]  InitialRot=[0 0 270]  ActorName=SimulinkVehicle35  SampleTime=-1  ActorType=SimulinkVehicle  ID=35  aMode=3  ActorTag=SimulinkVehicle35  CoordinateScheme=ISO  VehLightsControl=off  HeadlightColor=[ 1, 1, 1 ]  HighBeamIntensity=100000  LowBeamIntensity=60000  HighBeamConeAngle=70  LowBeamConeAngle=70  LeftHeadlightOrientation=[ 0, 0 ]  RightHeadlightOrientation=[ 0, 0 ]  BrakelightIntensity=500  ReverselightIntensity=500  SignallightIntensity=500  SignallightPeriod=1  SignalPulseWidth=50  TransformOutportEnabled=off
      settings: LibrarySourceBlock=drivingsim3d/Simulation 3D Vehicle with Ground Following
  vehicle35 : sim3dautolib/Simulation 3D Vehicle with Ground Following  Priority=-1  PassVehMesh=Hatchback  MeshPath=/MathWorksSimulation/Vehicles/Muscle/Meshes/SK_MuscleCar.SK_MuscleCar  TrackWidth=1.9  WheelBase=3  WheelRadius=0.35  VehColor=Yellow  InitialPos=[-10.42 53.21 0]  InitialRot=[0 0 90]  ActorName=SimulinkVehicle36  SampleTime=-1  ActorType=SimulinkVehicle  ID=36  aMode=3  ActorTag=SimulinkVehicle36  CoordinateScheme=ISO  VehLightsControl=off  HeadlightColor=[ 1, 1, 1 ]  HighBeamIntensity=100000  LowBeamIntensity=60000  HighBeamConeAngle=70  LowBeamConeAngle=70  LeftHeadlightOrientation=[ 0, 0 ]  RightHeadlightOrientation=[ 0, 0 ]  BrakelightIntensity=500  ReverselightIntensity=500  SignallightIntensity=500  SignallightPeriod=1  SignalPulseWidth=50  TransformOutportEnabled=off
      settings: LibrarySourceBlock=drivingsim3d/Simulation 3D Vehicle with Ground Following
  vehicle4 : sim3dautolib/Simulation 3D Vehicle with Ground Following  Priority=-1  PassVehMesh=Small pickup truck  MeshPath=/MathWorksSimulation/Vehicles/Muscle/Meshes/SK_MuscleCar.SK_MuscleCar  TrackWidth=1.9  WheelBase=3  WheelRadius=0.35  VehColor=White  InitialPos=[24.31 21.78 0]  InitialRot=[0 0 90]  ActorName=SimulinkVehicle5  SampleTime=-1  ActorType=SimulinkVehicle  ID=5  aMode=3  ActorTag=SimulinkVehicle5  CoordinateScheme=ISO  VehLightsControl=off  HeadlightColor=[ 1, 1, 1 ]  HighBeamIntensity=100000  LowBeamIntensity=60000  HighBeamConeAngle=70  LowBeamConeAngle=70  LeftHeadlightOrientation=[ 0, 0 ]  RightHeadlightOrientation=[ 0, 0 ]  BrakelightIntensity=500  ReverselightIntensity=500  SignallightIntensity=500  SignallightPeriod=1  SignalPulseWidth=50  TransformOutportEnabled=off
      settings: LibrarySourceBlock=drivingsim3d/Simulation 3D Vehicle with Ground Following
  vehicle5 : sim3dautolib/Simulation 3D Vehicle with Ground Following  Priority=-1  PassVehMesh=Sedan  MeshPath=/MathWorksSimulation/Vehicles/Muscle/Meshes/SK_MuscleCar.SK_MuscleCar  TrackWidth=1.9  WheelBase=3  WheelRadius=0.35  VehColor=Red  InitialPos=[19.37 21.59 0]  InitialRot=[0 0 270]  ActorName=SimulinkVehicle6  SampleTime=-1  ActorType=SimulinkVehicle  ID=6  aMode=3  ActorTag=SimulinkVehicle6  CoordinateScheme=ISO  VehLightsControl=off  HeadlightColor=[ 1, 1, 1 ]  HighBeamIntensity=100000  LowBeamIntensity=60000  HighBeamConeAngle=70  LowBeamConeAngle=70  LeftHeadlightOrientation=[ 0, 0 ]  RightHeadlightOrientation=[ 0, 0 ]  BrakelightIntensity=500  ReverselightIntensity=500  SignallightIntensity=500  SignallightPeriod=1  SignalPulseWidth=50  TransformOutportEnabled=off
      settings: LibrarySourceBlock=drivingsim3d/Simulation 3D Vehicle with Ground Following
  vehicle6 : sim3dautolib/Simulation 3D Vehicle with Ground Following  Priority=-1  PassVehMesh=Hatchback  MeshPath=/MathWorksSimulation/Vehicles/Muscle/Meshes/SK_MuscleCar.SK_MuscleCar  TrackWidth=1.9  WheelBase=3  WheelRadius=0.35  VehColor=Green  InitialPos=[13.89 21.59 0]  InitialRot=[0 0 90]  ActorName=SimulinkVehicle7  SampleTime=-1  ActorType=SimulinkVehicle  ID=7  aMode=3  ActorTag=SimulinkVehicle7  CoordinateScheme=ISO  VehLightsControl=off  HeadlightColor=[ 1, 1, 1 ]  HighBeamIntensity=100000  LowBeamIntensity=60000  HighBeamConeAngle=70  LowBeamConeAngle=70  LeftHeadlightOrientation=[ 0, 0 ]  RightHeadlightOrientation=[ 0, 0 ]  BrakelightIntensity=500  ReverselightIntensity=500  SignallightIntensity=500  SignallightPeriod=1  SignalPulseWidth=50  TransformOutportEnabled=off
      settings: LibrarySourceBlock=drivingsim3d/Simulation 3D Vehicle with Ground Following
  vehicle7 : sim3dautolib/Simulation 3D Vehicle with Ground Following  Priority=-1  PassVehMesh=Muscle car  MeshPath=/MathWorksSimulation/Vehicles/Muscle/Meshes/SK_MuscleCar.SK_MuscleCar  TrackWidth=1.9  WheelBase=3  WheelRadius=0.35  VehColor=Green  InitialPos=[11.15 21.59 0]  InitialRot=[0 0 90]  ActorName=SimulinkVehicle8  SampleTime=-1  ActorType=SimulinkVehicle  ID=8  aMode=3  ActorTag=SimulinkVehicle8  CoordinateScheme=ISO  VehLightsControl=off  HeadlightColor=[ 1, 1, 1 ]  HighBeamIntensity=100000  LowBeamIntensity=60000  HighBeamConeAngle=70  LowBeamConeAngle=70  LeftHeadlightOrientation=[ 0, 0 ]  RightHeadlightOrientation=[ 0, 0 ]  BrakelightIntensity=500  ReverselightIntensity=500  SignallightIntensity=500  SignallightPeriod=1  SignalPulseWidth=50  TransformOutportEnabled=off
      settings: LibrarySourceBlock=drivingsim3d/Simulation 3D Vehicle with Ground Following
  vehicle8 : sim3dautolib/Simulation 3D Vehicle with Ground Following  Priority=-1  PassVehMesh=Sport utility vehicle  MeshPath=/MathWorksSimulation/Vehicles/Muscle/Meshes/SK_MuscleCar.SK_MuscleCar  TrackWidth=1.9  WheelBase=3  WheelRadius=0.35  VehColor=Silver  InitialPos=[5.664 21.41 0]  InitialRot=[0 0 90]  ActorName=SimulinkVehicle9  SampleTime=-1  ActorType=SimulinkVehicle  ID=9  aMode=3  ActorTag=SimulinkVehicle9  CoordinateScheme=ISO  VehLightsControl=off  HeadlightColor=[ 1, 1, 1 ]  HighBeamIntensity=100000  LowBeamIntensity=60000  HighBeamConeAngle=70  LowBeamConeAngle=70  LeftHeadlightOrientation=[ 0, 0 ]  RightHeadlightOrientation=[ 0, 0 ]  BrakelightIntensity=500  ReverselightIntensity=500  SignallightIntensity=500  SignallightPeriod=1  SignalPulseWidth=50  TransformOutportEnabled=off
      settings: LibrarySourceBlock=drivingsim3d/Simulation 3D Vehicle with Ground Following
  vehicle9 : sim3dautolib/Simulation 3D Vehicle with Ground Following  Priority=-1  PassVehMesh=Small pickup truck  MeshPath=/MathWorksSimulation/Vehicles/Muscle/Meshes/SK_MuscleCar.SK_MuscleCar  TrackWidth=1.9  WheelBase=3  WheelRadius=0.35  VehColor=Silver  InitialPos=[2.74 21.41 0]  InitialRot=[0 0 270]  ActorName=SimulinkVehicle10  SampleTime=-1  ActorType=SimulinkVehicle  ID=10  aMode=3  ActorTag=SimulinkVehicle10  CoordinateScheme=ISO  VehLightsControl=off  HeadlightColor=[ 1, 1, 1 ]  HighBeamIntensity=100000  LowBeamIntensity=60000  HighBeamConeAngle=70  LowBeamConeAngle=70  LeftHeadlightOrientation=[ 0, 0 ]  RightHeadlightOrientation=[ 0, 0 ]  BrakelightIntensity=500  ReverselightIntensity=500  SignallightIntensity=500  SignallightPeriod=1  SignalPulseWidth=50  TransformOutportEnabled=off
      settings: LibrarySourceBlock=drivingsim3d/Simulation 3D Vehicle with Ground Following
  wires:
  Y34/1 -> vehicle34/2
  T35/1 -> vehicle35/3
  T34/1 -> vehicle34/3
  T16/1 -> vehicle16/3
  Y35/1 -> vehicle35/2
  T30/1 -> vehicle30/3
  Y11/1 -> vehicle11/2
  X35/1 -> vehicle35/1
  Y33/1 -> vehicle33/2
  T11/1 -> vehicle11/3
  T22/1 -> vehicle22/3
  X34/1 -> vehicle34/1
  T33/1 -> vehicle33/3
  Y16/1 -> vehicle16/2
  T24/1 -> vehicle24/3
  X33/1 -> vehicle33/1
  T32/1 -> vehicle32/3
  Y21/1 -> vehicle21/2
  Y32/1 -> vehicle32/2
  X22/1 -> vehicle22/1
  T6/1 -> vehicle6/3
  X12/1 -> vehicle12/1
  X32/1 -> vehicle32/1
  Y14/1 -> vehicle14/2
  T31/1 -> vehicle31/3
  T18/1 -> vehicle18/3
  X20/1 -> vehicle20/1
  Y31/1 -> vehicle31/2
  X31/1 -> vehicle31/1
  T26/1 -> vehicle26/3
  X28/1 -> vehicle28/1
  Y25/1 -> vehicle25/2
  Y30/1 -> vehicle30/2
  X30/1 -> vehicle30/1
  T29/1 -> vehicle29/3
  Y29/1 -> vehicle29/2
  T1/1 -> vehicle1/3
  T19/1 -> vehicle19/3
  X29/1 -> vehicle29/1
  T28/1 -> vehicle28/3
  Y23/1 -> vehicle23/2
  Y28/1 -> vehicle28/2
  X19/1 -> vehicle19/1
  T27/1 -> vehicle27/3
  Y27/1 -> vehicle27/2
  T20/1 -> vehicle20/3
  Y15/1 -> vehicle15/2
  X27/1 -> vehicle27/1
  Y26/1 -> vehicle26/2
  T15/1 -> vehicle15/3
  X17/1 -> vehicle17/1
  X26/1 -> vehicle26/1
  X16/1 -> vehicle16/1
  T25/1 -> vehicle25/3
  Y20/1 -> vehicle20/2
  X25/1 -> vehicle25/1
  Y24/1 -> vehicle24/2
  T14/1 -> vehicle14/3
  X24/1 -> vehicle24/1
  T23/1 -> vehicle23/3
  X23/1 -> vehicle23/1
  Y22/1 -> vehicle22/2
  T21/1 -> vehicle21/3
  X21/1 -> vehicle21/1
  Y19/1 -> vehicle19/2
  Y18/1 -> vehicle18/2
  Y17/1 -> vehicle17/2
  X18/1 -> vehicle18/1
  X15/1 -> vehicle15/1
  T17/1 -> vehicle17/3
  X14/1 -> vehicle14/1
  T13/1 -> vehicle13/3
  Y13/1 -> vehicle13/2
  X13/1 -> vehicle13/1
  T12/1 -> vehicle12/3
  Y12/1 -> vehicle12/2
  X11/1 -> vehicle11/1
  T10/1 -> vehicle10/3
  Y10/1 -> vehicle10/2
  X3/1 -> vehicle3/1
  X10/1 -> vehicle10/1
  T9/1 -> vehicle9/3
  Y9/1 -> vehicle9/2
  X9/1 -> vehicle9/1
  T8/1 -> vehicle8/3
  Y8/1 -> vehicle8/2
  X8/1 -> vehicle8/1
  T7/1 -> vehicle7/3
  Y7/1 -> vehicle7/2
  X7/1 -> vehicle7/1
  Y6/1 -> vehicle6/2
  X6/1 -> vehicle6/1
  T5/1 -> vehicle5/3
  Y5/1 -> vehicle5/2
  X5/1 -> vehicle5/1
  T4/1 -> vehicle4/3
  Y4/1 -> vehicle4/2
  X4/1 -> vehicle4/1
  T3/1 -> vehicle3/3
  Y3/1 -> vehicle3/2
  T2/1 -> vehicle2/3
  Y2/1 -> vehicle2/2
  X2/1 -> vehicle2/1
  Y1/1 -> vehicle1/2
  X1/1 -> vehicle1/1

== matlab function localizeUsingLidar/MATLAB Function ==
  data: lidarEstX output; xyzPoints input; lidarEstY output; lidarEstYaw output; loc input; or input; mapPoints input
function [lidarEstX,lidarEstY,lidarEstYaw] = Localize(xyzPoints,loc,or,mapPoints)
    
    persistent initPose frameCount ndtMap;
    coder.extrinsic("helperLidarLocalizerNDT","pcmapndt","pointCloud","selectSubmap","rigid3d");
    submapSize = [30 30 5];  
    
    % Create ndt map from point cloud map at the beginning of simulation
    if isempty(ndtMap)
        rng(0)
        ptMap = pointCloud(mapPoints);
        ndtMap = pcmapndt(ptMap,1);
    end
    
    % select submap region using the initial pose estimate
    if isempty(frameCount)
        frameCount = 0; 
        ndtMap = selectSubmap(ndtMap,loc,submapSize);
        lidarEstYaw = or(3);
        rot = [cos(lidarEstYaw), sin(lidarEstYaw),  0; ...
        -sin(lidarEstYaw), cos(lidarEstYaw), 0; ...
        0,         0,    1];
        initPose = rigid3d(single(rot),single(loc));
    else
        frameCount = frameCount + 1;
    end
    
    % Localize and find pose estimate
    hasNoPoints = all( isnan(xyzPoints), 'all' );
    if hasNoPoints
        lidarEstX   = single(NaN);
        lidarEstY   = single(NaN);
        lidarEstYaw = single(NaN);
        return;
    else
        [ndtMap,lidarEstX,lidarEstY,lidarEstYaw,initPose] = helperLidarLocalizerNDT(xyzPoints,ndtMap,initPose);
    end
end

== matlab function localizeUsingLidar/MATLAB Function1 ==
  data: gTruthLocation input; lidarEstX input; lidarEstY input; lidarEstYaw input
function VisualizeLocalization(gTruthLocation,lidarEstX,lidarEstY,lidarEstYaw)
%VisualizeLocalizationPath Visualize localization path.

coder.extrinsic('helperGetSceneImage', 'figure', 'imshow', 'title', ...
    'get', 'set', 'movegui', 'gca', 'isvalid', 'hold','showShape', 'scatter', ...
    'helperUpdateScatter', 'xlim', 'ylim','legend');

persistent hFig hAx hScEst hScGt;

vehicleColor = [0.85 0.325 0.098];
vehicleDims  = [3.864 1.960];
markerSize   = 8;

gX = gTruthLocation(1);
gY = gTruthLocation(2);

if isempty(hFig)
    % Query the model to find the scene selection
    sceneName = 'LargeParkingLot';
    [sceneImage, sceneRef] = helperGetSceneImage(sceneName);
    
    % Create a figure and display the scene on it
    hFig = figure('Name', 'Scene Map Display');
    hIm = imshow(sceneImage, sceneRef, 'InitialMagnification', 12.5);
    hAx  = get(hIm,'Parent');
    set(hAx, 'YDir', 'normal');
    title(hAx, 'Localization estimate using an NDT map');
    xlim(hAx, [-60 40]);
    ylim(hAx, [10 60]);
    
    hold(hAx, 'on')
    hScGt = scatter(hAx, NaN, NaN, 10, [0 1 0], '*');
    hScEst = scatter(hAx, NaN, NaN, markerSize, vehicleColor, 'filled');  
    legend("Estimated Position","Ground Truth Position");
    hold(hAx, 'off')
    
    % Move figure to right of screen
    movegui(hFig, 'east');
end

if isvalid(hFig) && isfinite(lidarEstX) && isfinite(lidarEstY) && isfinite(lidarEstYaw)
    showShape('rectangle', [lidarEstX lidarEstY vehicleDims rad2deg(lidarEstYaw)], ...
        'Parent', hAx, 'Color', vehicleColor, 'Opacity', 0.2);
    
    helperUpdateScatter(hScGt, gX, gY);
    helperUpdateScatter(hScEst, lidarEstX, lidarEstY);
    
    k = 1;
    
end
end
